simulink model "voltage"  (R2024b)
settings: Solver=VariableStepAuto  StartTime=0.0  StopTime=10.0  RelTol=1e-3
settings Model: Creator=10537  LastModifiedBy=10537

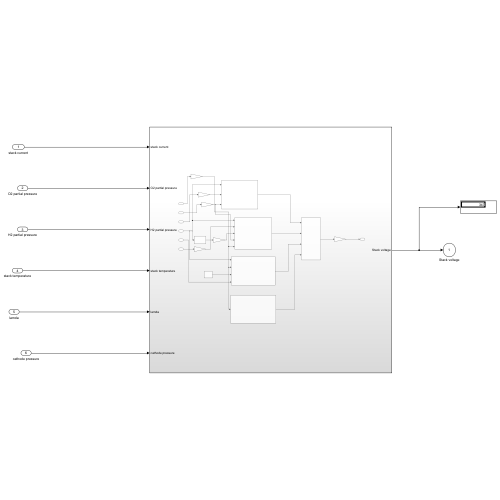
[thumbnail: Simulink's stored preview of the top-level diagram]
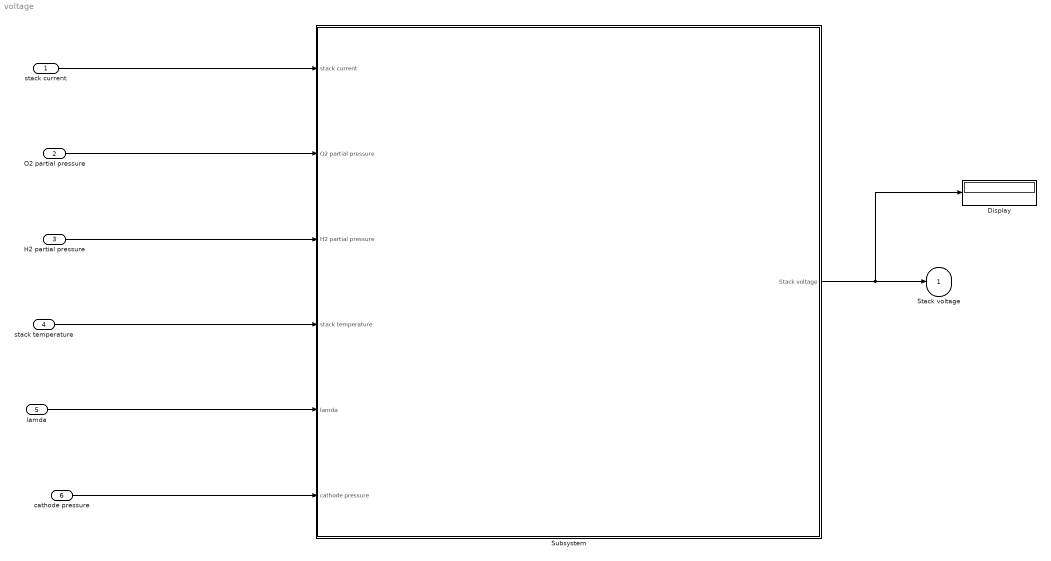
== system voltage ==
  stack current : Inport
  O2 partial pressure : Inport  Port=2
  H2 partial pressure : Inport  Port=3
  stack temperature : Inport  Port=4
  lamda : Inport  Port=5
  cathode pressure : Inport  Port=6
  Display : Display
  Subsystem : Subsystem
  Stack voltage : Outport
  wires:
  Subsystem/1(Stack voltage) -> Display/1, Stack voltage/1
  stack current/1 -> Subsystem/1(stack current)
  O2 partial pressure/1 -> Subsystem/2(O2 partial pressure)
  H2 partial pressure/1 -> Subsystem/3(H2 partial pressure)
  stack temperature/1 -> Subsystem/4(stack temperature)
  lamda/1 -> Subsystem/5(lamda)
  cathode pressure/1 -> Subsystem/6(cathode pressure)

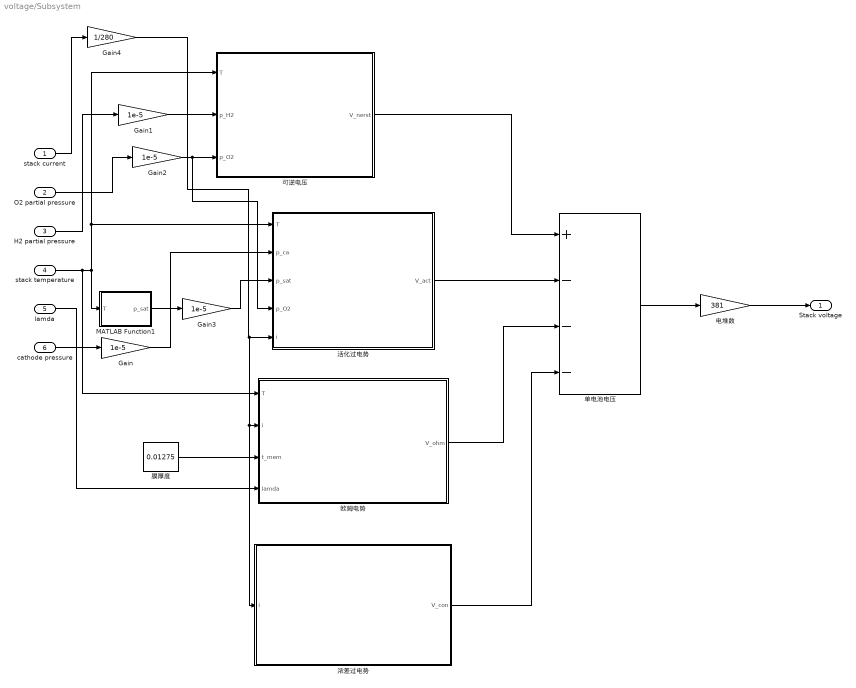
== system voltage/Subsystem ==
  stack current : Inport
  O2 partial pressure : Inport  Port=2
  H2 partial pressure : Inport  Port=3
  stack temperature : Inport  Port=4
  lamda : Inport  Port=5
  cathode pressure : Inport  Port=6
  Gain{,1..3} (4 alike) : Gain  Gain=1e-5
  Gain4 : Gain  Gain=1/280
  MATLAB Function1 : MATLAB Function  TreatAsAtomicUnit=on
  单电池电压 : Sum  Inputs=+---
  可逆电压 : MATLAB Function  TreatAsAtomicUnit=on
  欧姆电势 : MATLAB Function  TreatAsAtomicUnit=on
  活化过电势 : MATLAB Function  TreatAsAtomicUnit=on
  "浓差过电势 " : MATLAB Function  TreatAsAtomicUnit=on
  电堆数 : Gain  Gain=381
  膜厚度 : Constant  Value=0.01275
  Stack voltage : Outport
  wires:
  stack temperature/1 -> 欧姆电势/1(T), MATLAB Function1/1(T), 活化过电势/1(T), 可逆电压/1(T)
  O2 partial pressure/1 -> Gain2/1
  cathode pressure/1 -> Gain/1
  H2 partial pressure/1 -> Gain1/1
  膜厚度/1 -> 欧姆电势/3(t_mem)
  stack current/1 -> Gain4/1
  Gain2/1 -> 活化过电势/4(p_O2), 可逆电压/3(p_O2)
  Gain4/1 -> "浓差过电势 "/1(i), 欧姆电势/2(i), 活化过电势/5(i)
  单电池电压/1 -> 电堆数/1
  MATLAB Function1/1(p_sat) -> Gain3/1
  Gain3/1 -> 活化过电势/3(p_sat)
  "浓差过电势 "/1(V_con) -> 单电池电压/4
  lamda/1 -> 欧姆电势/4(lamda)
  Gain/1 -> 活化过电势/2(p_ca)
  可逆电压/1(V_nerst) -> 单电池电压/1
  电堆数/1 -> Stack voltage/1
  活化过电势/1(V_act) -> 单电池电压/2
  Gain1/1 -> 可逆电压/2(p_H2)
  欧姆电势/1(V_ohm) -> 单电池电压/3

== matlab function voltage/Subsystem/活化过电势 ==
  data: T input; V_act output; p_ca input; p_sat input; p_O2 input; i input
function V_act = fcn(T,p_ca,p_sat,p_O2,i)

V0=0.279-8.5e-4*(T-298.15)+4.308e-4*T*(log((p_ca-p_sat)/1.01325)+0.5*log(0.1173*(p_ca-p_sat)/1.01325));
Va = (-1.618e-5*T+1.618e-2)*(p_O2/0.1173+p_sat)^2+(1.8e-4*T-0.166)*(p_O2/0.1173+p_sat)+(-5.8e-4*T+0.5736);
c=10;
V_act = V0+Va*(1-exp(-c*i));

== matlab function voltage/Subsystem/可逆电压 ==
  data: T input; V_nerst output; p_H2 input; p_O2 input
function V_nerst= fcn(T,p_H2,p_O2)

V_nerst = 1.229-8.5e-4*(T-298.15)+4.3085e-5*T*(log(p_H2)+0.5*log(p_O2));

== matlab function voltage/Subsystem/MATLAB Function1 ==
  data: T input; p_sat output
function p_sat = fcn(T)

p_sat = exp(23.196-3816.44/ (T-46.13));

== matlab function voltage/Subsystem/欧姆电势 ==
  data: T input; V_ohm output; i input; t_mem input; lamda input
function V_ohm = fcn(T,i,t_mem,lamda)

sigma=(0.514*lamda-0.033)*exp(1268*(1/303-1/T));
R_ohm=t_mem/sigma;
V_ohm = i*R_ohm;

== matlab function voltage/Subsystem/浓差过电势  ==
  data: i input; V_con output
function V_con = fcn(i)

V_con = 0.016*log(1.5/(1.5-i));
